simulink model "VSRMathematicalModel"  (R2021a)
settings: Solver=VariableStepAuto  StartTime=0.0  StopTime=0.3  FixedStep=5e-6  MaxStep=1e-6  RelTol=1e-3
InitFcn:
  | L = 2e-3;
  | omega = 2*pi*50;
  | a = exp(1i*2*pi/3);
  | R = 0.5;
  | C  = 1000e-6;
  | tau_c = 1.6e-4;
  | kp = L/tau_c;
  | ki = R/tau_c;
undefined symbols (not defined in the file): DiscIntNeverNeededParam
libraries: pid_lib x4
settings Model: Creator=Kibrom  LastModifiedBy=Kibrom

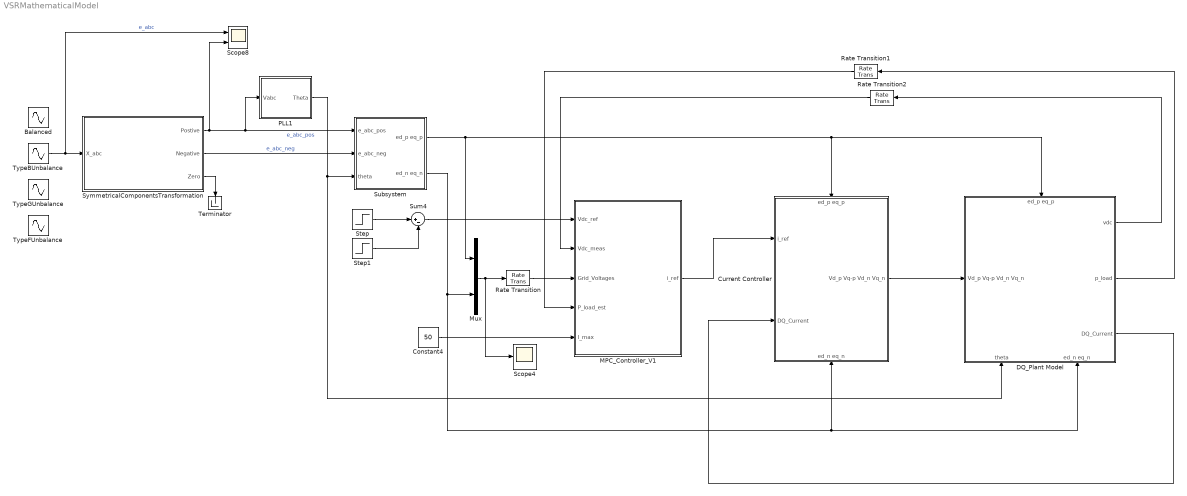
== system VSRMathematicalModel ==
  Balanced : Sin  Amplitude=sqrt(2)*[230 230 230]  Frequency=2*pi*50  Phase=[0 240 120]*(pi/180)  SampleTime=1e-4
  Constant4 : Constant  Value=50  SampleTime=1e-3
  Current Controller : Subsystem
      settings: PortSchema="{\"entries\":[{\"content\":{\"sides\":[{\"content\":{\"connectorIds\":[\"In1\",\"In2\"]},\"type\":\"ConnectorPlacement.EquallySpacedRectSide\",\"uuid\":\"d43164cf-c134-48fd-af5b-783b7be86266\"},{\"content\":{\"connectorIds\":[\"Out1\"],\"side\":\"RIGHT\"},\"type\":\"ConnectorPlacement.EquallySpacedRectSide\",\"uuid\":\"14eb066f-1df9-45e9-95e8-1c3f6be4e42a\"},{\"content\":{\"connectorIds\":[\"In3\"],\"side\":\"TOP\"},\"type\":\"ConnectorPlacement.EquallySpacedRectSide\",\"uuid\":\"0a2a25ed-4570-4f3f-83bf-cfa199df058c\"},{\"content\":{\"connectorIds\":[\"In4\"],\"side\":\"BOTTOM\"},\"type\":\"ConnectorPlacement.EquallySpacedRectSide\",\"uuid\":\"5d5e5ab5-6582-423d-8129-1371a7fc0364\"}]},\"type\":\"ConnectorPlacement.EquallySpacedConnector\",\"uuid\":\"cd9b7e71-8f1f-4781-be87-4737fe6c2517\"}],\"packageUris\":[\"http://schema.mathworks.com/mf0/Connector/R2020b\"],\"version\":\"1.0\"}"
  DQ_Plant Model : Subsystem
      settings: PortSchema="{\"entries\":[{\"content\":{\"sides\":[{\"content\":{\"connectorIds\":[\"In1\"]},\"type\":\"ConnectorPlacement.EquallySpacedRectSide\",\"uuid\":\"562d4ce7-556e-457d-bc10-9586690b759c\"},{\"content\":{\"connectorIds\":[\"Out1\",\"Out2\",\"Out3\"],\"side\":\"RIGHT\"},\"type\":\"ConnectorPlacement.EquallySpacedRectSide\",\"uuid\":\"d4e8a128-6870-4c36-a811-937c88534be6\"},{\"content\":{\"connectorIds\":[\"In2\"],\"side\":\"TOP\"},\"type\":\"ConnectorPlacement.EquallySpacedRectSide\",\"uuid\":\"ff397437-20b8-4b49-bf3a-8efc1e28b27f\"},{\"content\":{\"connectorIds\":[\"In3\",\"In4\"],\"side\":\"BOTTOM\"},\"type\":\"ConnectorPlacement.EquallySpacedRectSide\",\"uuid\":\"84aa63e1-bec8-4c80-97ac-aae86762ebfb\"}]},\"type\":\"ConnectorPlacement.EquallySpacedConnector\",\"uuid\":\"64a36633-d751-446b-85f3-9153f3d81120\"}],\"packageUris\":[\"http://schema.mathworks.com/mf0/Connector/R2020b\"],\"version\":\"1.0\"}"
  MPC_Controller_V1 : MATLAB Function  TreatAsAtomicUnit=on  SystemSampleTime=1e-3
  Mux : Mux  Inputs=2
  PLL1 : Subsystem
  Rate Transition : RateTransition  OutPortSampleTime=1000e-6
  Rate Transition1 : RateTransition
  Rate Transition2 : RateTransition
  Scope4 : Scope
  Scope8 : Scope  NumInputPorts=2
  Step : Step  Time=0.1  Before=650  After=750  SampleTime=1e-3
  Step1 : Step  Time=0.2  After=50  SampleTime=1e-3
  Subsystem : Subsystem
  Sum4 : Sum  Inputs=|+-
  SymmetricalComponentsTransformation : Subsystem
  Terminator : Terminator
  TypeBUnbalance : Sin  Amplitude=sqrt(2)*[185 230 230]  Frequency=2*pi*50  Phase=[0 240 120]*(pi/180)  SampleTime=0
  TypeFUnbalance : Sin  Amplitude=sqrt(2)*[184 207.4 207.4]  Frequency=2*pi*50  Phase=[0 243.7 116.3]*(pi/180)  SampleTime=0
  TypeGUnbalance : Sin  Amplitude=sqrt(2)*[214.6 192.1 192.1]  Frequency=2*pi*50  Phase=[0 236 124]*(pi/180)  SampleTime=0
  wires:
  SymmetricalComponentsTransformation/3(Zero) -> Terminator/1
  TypeBUnbalance/1 -> Scope8/1, SymmetricalComponentsTransformation/1(X_abc)  "e_abc"
  MPC_Controller_V1/1(i_ref) -> Current Controller/1(i_ref)
  Step/1 -> Sum4/1
  Mux/1 -> Scope4/1, Rate Transition/1
  Constant4/1 -> MPC_Controller_V1/5(I_max)
  Rate Transition/1 -> MPC_Controller_V1/3(Grid_Voltages)
  Rate Transition1/1 -> MPC_Controller_V1/4(P_load_est)
  Rate Transition2/1 -> MPC_Controller_V1/2(Vdc_meas)
  Step1/1 -> Sum4/2
  Sum4/1 -> MPC_Controller_V1/1(Vdc_ref)
  PLL1/1(Theta) -> Subsystem/3(theta), DQ_Plant Model/3(theta)
  SymmetricalComponentsTransformation/1(Postive) -> Scope8/2, Subsystem/1(e_abc_pos), PLL1/1(Vabc)  "e_abc_pos"
  Current Controller/1(Vd_p Vq-p Vd_n Vq_n) -> DQ_Plant Model/1(Vd_p Vq-p Vd_n Vq_n)
  DQ_Plant Model/1(vdc) -> Rate Transition2/1
  DQ_Plant Model/2(p_load) -> Rate Transition1/1
  DQ_Plant Model/3(DQ_Current) -> Current Controller/2(DQ_Current)
  Subsystem/1(ed_p eq_p) -> Mux/1, Current Controller/3(ed_p eq_p), DQ_Plant Model/2(ed_p eq_p)
  Subsystem/2(ed_n eq_n) -> Current Controller/4(ed_n eq_n), DQ_Plant Model/4(ed_n eq_n), Mux/2
  SymmetricalComponentsTransformation/2(Negative) -> Subsystem/2(e_abc_neg)  "e_abc_neg"

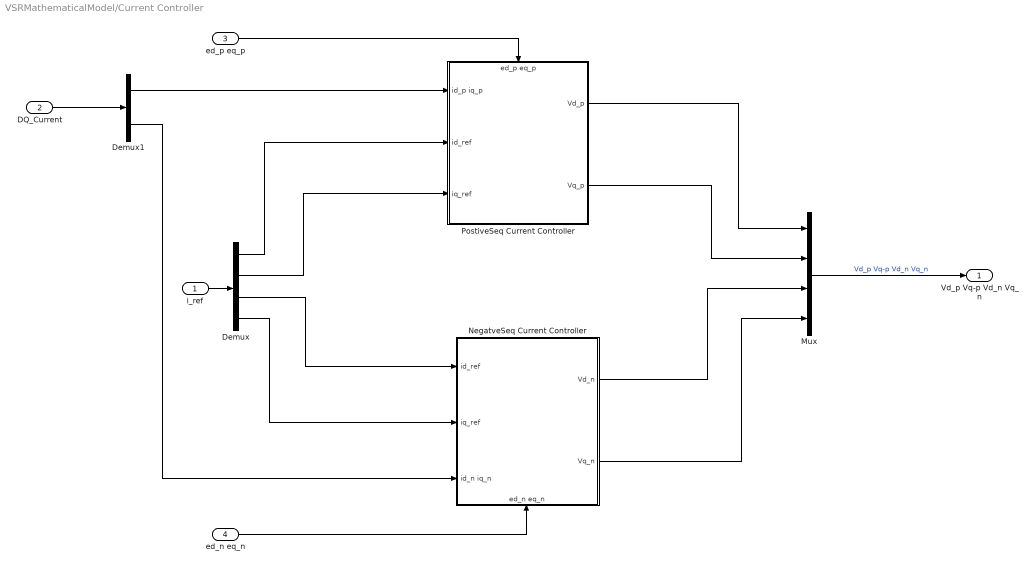
== system VSRMathematicalModel/Current Controller ==
  i_ref : Inport
  DQ_Current : Inport  Port=2
  ed_p eq_p : Inport  Port=3
  ed_n eq_n : Inport  Port=4
  Demux : Demux
  Demux1 : Demux  Outputs=2
  Mux : Mux
  NegatveSeq Current Controller : Subsystem
      settings: PortSchema="{\"entries\":[{\"content\":{\"sides\":[{\"content\":{\"connectorIds\":[\"In1\",\"In2\",\"In3\"]},\"type\":\"ConnectorPlacement.EquallySpacedRectSide\",\"uuid\":\"2bdf4aa8-c3f9-436b-9835-043d932fea71\"},{\"content\":{\"connectorIds\":[\"Out1\",\"Out2\"],\"side\":\"RIGHT\"},\"type\":\"ConnectorPlacement.EquallySpacedRectSide\",\"uuid\":\"c965a7a2-5936-47cc-8492-850bd324378e\"},{\"content\":{\"connectorIds\":[],\"side\":\"TOP\"},\"type\":\"ConnectorPlacement.EquallySpacedRectSide\",\"uuid\":\"45debca4-d3b7-48eb-be8d-4eccd646cb24\"},{\"content\":{\"connectorIds\":[\"In4\"],\"side\":\"BOTTOM\"},\"type\":\"ConnectorPlacement.EquallySpacedRectSide\",\"uuid\":\"6975aea9-83b3-4c6b-a4f1-94e60a0e1fe9\"}]},\"type\":\"ConnectorPlacement.EquallySpacedConnector\",\"uuid\":\"b897b5d1-f6c9-41b8-aee6-e6cc6417929b\"}],\"packageUris\":[\"http://schema.mathworks.com/mf0/Connector/R2020b\"],\"version\":\"1.0\"}"
  PostiveSeq Current Controller : Subsystem
      settings: PortSchema="{\"entries\":[{\"content\":{\"sides\":[{\"content\":{\"connectorIds\":[\"In1\",\"In2\",\"In3\"]},\"type\":\"ConnectorPlacement.EquallySpacedRectSide\",\"uuid\":\"2bdf4aa8-c3f9-436b-9835-043d932fea71\"},{\"content\":{\"connectorIds\":[\"Out1\",\"Out2\"],\"side\":\"RIGHT\"},\"type\":\"ConnectorPlacement.EquallySpacedRectSide\",\"uuid\":\"c965a7a2-5936-47cc-8492-850bd324378e\"},{\"content\":{\"connectorIds\":[\"In4\"],\"side\":\"TOP\"},\"type\":\"ConnectorPlacement.EquallySpacedRectSide\",\"uuid\":\"45debca4-d3b7-48eb-be8d-4eccd646cb24\"}]},\"type\":\"ConnectorPlacement.EquallySpacedConnector\",\"uuid\":\"b897b5d1-f6c9-41b8-aee6-e6cc6417929b\"}],\"packageUris\":[\"http://schema.mathworks.com/mf0/Connector/R2020b\"],\"version\":\"1.0\"}"
  Vd_p Vq-p Vd_n Vq_n : Outport
  wires:
  Demux1/1 -> PostiveSeq Current Controller/1(id_p iq_p)
  Demux/3 -> NegatveSeq Current Controller/1(id_ref)
  ed_n eq_n/1 -> NegatveSeq Current Controller/4(ed_n eq_n)
  PostiveSeq Current Controller/1(Vd_p) -> Mux/1
  ed_p eq_p/1 -> PostiveSeq Current Controller/4(ed_p eq_p)
  Demux/4 -> NegatveSeq Current Controller/2(iq_ref)
  NegatveSeq Current Controller/1(Vd_n) -> Mux/3
  NegatveSeq Current Controller/2(Vq_n) -> Mux/4
  Demux/1 -> PostiveSeq Current Controller/2(id_ref)
  Demux/2 -> PostiveSeq Current Controller/3(iq_ref)
  PostiveSeq Current Controller/2(Vq_p) -> Mux/2
  Demux1/2 -> NegatveSeq Current Controller/3(id_n iq_n)
  Mux/1 -> Vd_p Vq-p Vd_n Vq_n/1  "Vd_p Vq-p Vd_n Vq_n"
  i_ref/1 -> Demux/1
  DQ_Current/1 -> Demux1/1

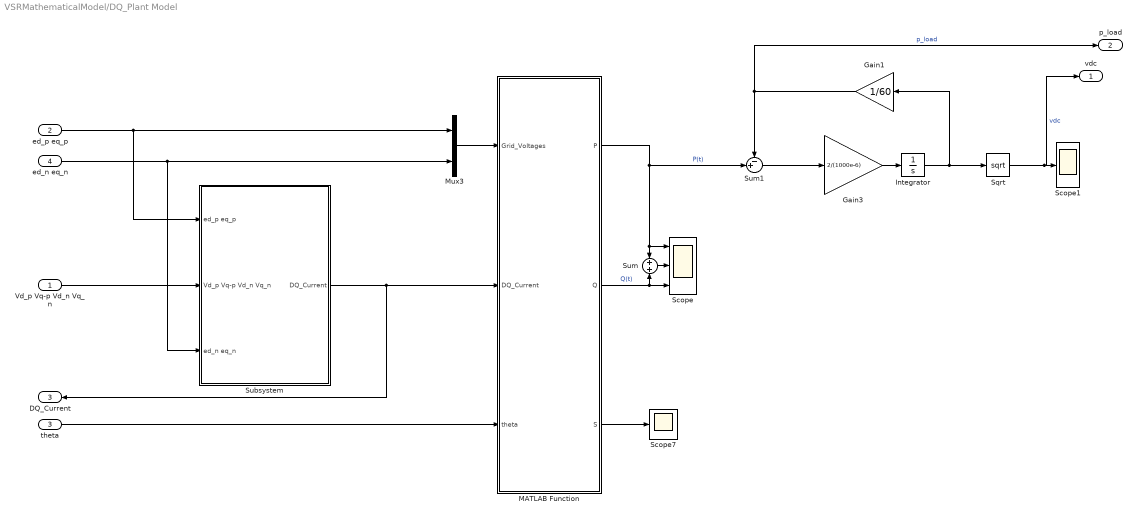
== system VSRMathematicalModel/DQ_Plant Model ==
  Vd_p Vq-p Vd_n Vq_n : Inport
  ed_p eq_p : Inport  Port=2
  theta : Inport  Port=3
  ed_n eq_n : Inport  Port=4
  Gain1 : Gain  Gain=1/60
  Gain3 : Gain  Gain=2/(1000e-6)
  Integrator : Integrator  InitialCondition=(650)^2
  MATLAB Function : MATLAB Function  TreatAsAtomicUnit=on
  Mux3 : Mux  Inputs=2
  Scope : Scope  NumInputPorts=3
  Scope1 : Scope
  Scope7 : Scope
  Sqrt : Sqrt  SaturateOnIntegerOverflow=on
  Subsystem : Subsystem
  Sum : Sum
  Sum1 : Sum  Inputs=-+|
  vdc : Outport
  p_load : Outport  Port=2
  DQ_Current : Outport  Port=3
  wires:
  MATLAB Function/3(S) -> Scope7/1
  Integrator/1 -> Sqrt/1, Gain1/1
  Gain1/1 -> p_load/1, Sum1/1  "p_load"
  ed_p eq_p/1 -> Subsystem/1(ed_p eq_p), Mux3/1
  MATLAB Function/2(Q) -> Scope/3, Sum/2  "Q(t)"
  Sum/1 -> Scope/2
  Gain3/1 -> Integrator/1
  MATLAB Function/1(P) -> Sum1/2, Scope/1, Sum/1  "P(t)"
  Sum1/1 -> Gain3/1
  Sqrt/1 -> vdc/1, Scope1/1  "vdc"
  ed_n eq_n/1 -> Subsystem/3(ed_n eq_n), Mux3/2
  Mux3/1 -> MATLAB Function/1(Grid_Voltages)
  Subsystem/1(DQ_Current) -> DQ_Current/1, MATLAB Function/2(DQ_Current)
  theta/1 -> MATLAB Function/3(theta)
  Vd_p Vq-p Vd_n Vq_n/1 -> Subsystem/2(Vd_p Vq-p Vd_n Vq_n)

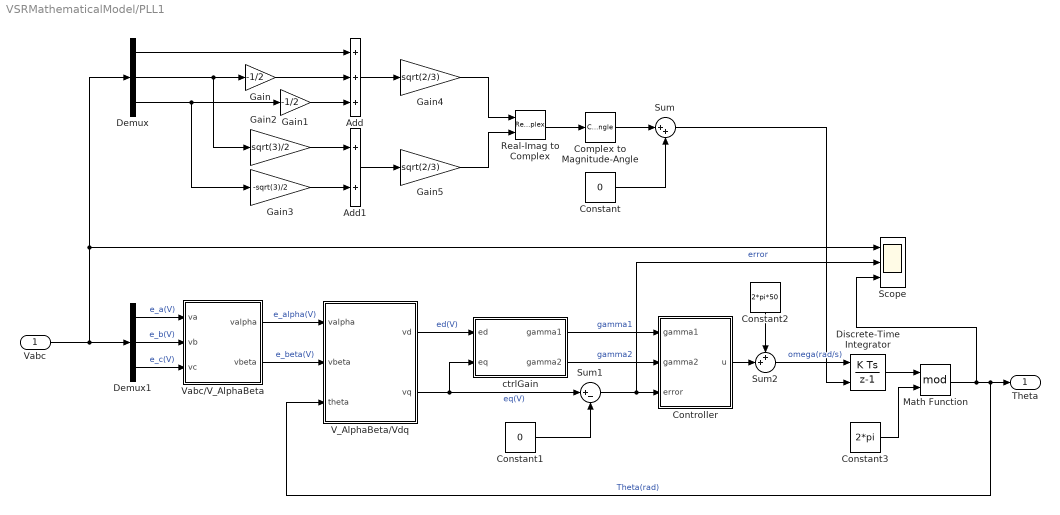
== system VSRMathematicalModel/PLL1 ==
  Vabc : Inport
  Add : Sum  Inputs=+++
  Add1 : Sum
  Complex to Magnitude-Angle : ComplexToMagnitudeAngle  Output=Angle
  Constant : Constant  Value=0
  Constant1 : Constant  Value=0
  Constant2 : Constant  Value=2*pi*50
  Constant3 : Constant  Value=2*pi
  Controller : Subsystem
  Demux : Demux  Outputs=3
  Demux1 : Demux  Outputs=3
  Discrete-Time Integrator : DiscreteIntegrator  InitialConditionSource=external  SampleTime=1e-4  ICPrevOutput=DiscIntNeverNeededParam  ICPrevScaledInput=DiscIntNeverNeededParam
  Gain : Gain  Gain=-1/2
  Gain1 : Gain  Gain=-1/2
  Gain2 : Gain  Gain=sqrt(3)/2
  Gain3 : Gain  Gain=-sqrt(3)/2
  Gain4 : Gain  Gain=sqrt(2/3)
  Gain5 : Gain  Gain=sqrt(2/3)
  Math Function : Math  Operator=mod  SaturateOnIntegerOverflow=on
  Real-Imag to Complex : RealImagToComplex
  Scope : Scope  NumInputPorts=3
  Sum : Sum  Inputs=|++
  Sum1 : Sum  Inputs=|+-
  Sum2 : Sum  Inputs=++|
  V_AlphaBeta/Vdq : MATLAB Function  TreatAsAtomicUnit=on
  Vabc/V_AlphaBeta : MATLAB Function  TreatAsAtomicUnit=on
  ctrlGain : MATLAB Function  TreatAsAtomicUnit=on
  Theta : Outport
  wires:
  Demux/2 -> Gain/1, Gain2/1
  Gain5/1 -> Real-Imag to Complex/2
  Add/1 -> Gain4/1
  Demux/3 -> Gain1/1, Gain3/1
  Gain/1 -> Add/2
  Gain4/1 -> Real-Imag to Complex/1
  Gain3/1 -> Add1/2
  Demux/1 -> Add/1
  Real-Imag to Complex/1 -> Complex to Magnitude-Angle/1
  Gain1/1 -> Add/3
  Add1/1 -> Gain5/1
  Gain2/1 -> Add1/1
  Complex to Magnitude-Angle/1 -> Sum/1
  Sum/1 -> Discrete-Time Integrator/2
  Constant/1 -> Sum/2
  Demux1/2 -> Vabc/V_AlphaBeta/2(vb)  "e_b(V)"
  Demux1/3 -> Vabc/V_AlphaBeta/3(vc)  "e_c(V)"
  Demux1/1 -> Vabc/V_AlphaBeta/1(va)  "e_a(V)"
  Vabc/V_AlphaBeta/2(vbeta) -> V_AlphaBeta/Vdq/2(vbeta)  "e_beta(V)"
  Vabc/V_AlphaBeta/1(valpha) -> V_AlphaBeta/Vdq/1(valpha)  "e_alpha(V)"
  V_AlphaBeta/Vdq/2(vq) -> ctrlGain/2(eq), Sum1/1  "eq(V)"
  Constant1/1 -> Sum1/2
  Constant2/1 -> Sum2/1
  Sum2/1 -> Discrete-Time Integrator/1  "omega(rad/s)"
  Discrete-Time Integrator/1 -> Math Function/1
  V_AlphaBeta/Vdq/1(vd) -> ctrlGain/1(ed)  "ed(V)"
  ctrlGain/1(gamma1) -> Controller/1(gamma1)  "gamma1"
  ctrlGain/2(gamma2) -> Controller/2(gamma2)  "gamma2"
  Sum1/1 -> Scope/2, Controller/3(error)  "error"
  Controller/1(u) -> Sum2/2
  Math Function/1 -> Scope/3, Theta/1, V_AlphaBeta/Vdq/3(theta)  "Theta(rad)"
  Constant3/1 -> Math Function/2
  Vabc/1 -> Demux/1, Scope/1, Demux1/1

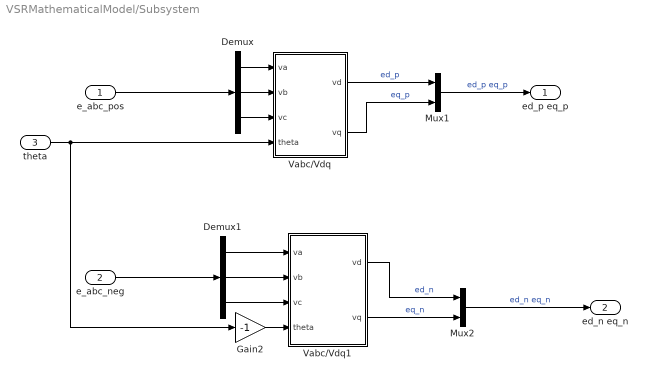
== system VSRMathematicalModel/Subsystem ==
  e_abc_pos : Inport
  e_abc_neg : Inport  Port=2
  theta : Inport  Port=3
  Demux : Demux  Outputs=3
  Demux1 : Demux  Outputs=3
  Gain2 : Gain  Gain=-1
  Mux1 : Mux  Inputs=2
  Mux2 : Mux  Inputs=2
  Vabc/Vdq : MATLAB Function  TreatAsAtomicUnit=on
  Vabc/Vdq1 : MATLAB Function  TreatAsAtomicUnit=on
  ed_p eq_p : Outport
  ed_n eq_n : Outport  Port=2
  wires:
  Vabc/Vdq1/2(vq) -> Mux2/2  "eq_n"
  Demux/1 -> Vabc/Vdq/1(va)
  Vabc/Vdq/1(vd) -> Mux1/1  "ed_p"
  Demux/2 -> Vabc/Vdq/2(vb)
  Demux1/3 -> Vabc/Vdq1/3(vc)
  Vabc/Vdq1/1(vd) -> Mux2/1  "ed_n"
  Demux1/2 -> Vabc/Vdq1/2(vb)
  Vabc/Vdq/2(vq) -> Mux1/2  "eq_p"
  e_abc_pos/1 -> Demux/1
  Demux1/1 -> Vabc/Vdq1/1(va)
  Gain2/1 -> Vabc/Vdq1/4(theta)
  Demux/3 -> Vabc/Vdq/3(vc)
  Mux1/1 -> ed_p eq_p/1  "ed_p eq_p"
  Mux2/1 -> ed_n eq_n/1  "ed_n eq_n"
  theta/1 -> Gain2/1, Vabc/Vdq/4(theta)
  e_abc_neg/1 -> Demux1/1

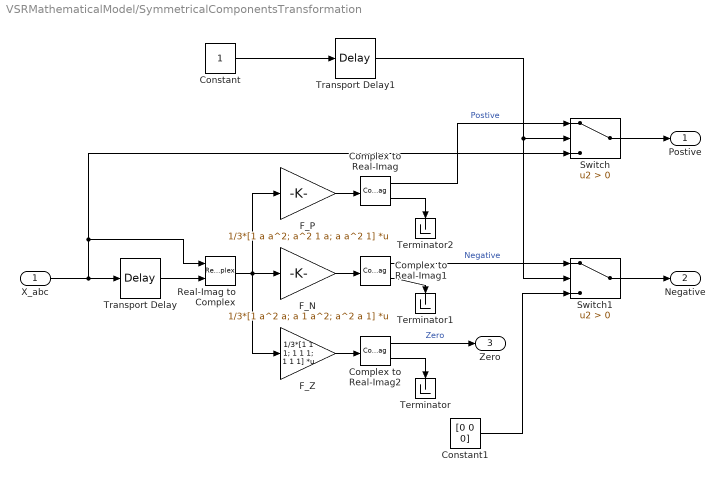
== system VSRMathematicalModel/SymmetricalComponentsTransformation ==
  X_abc : Inport
  Complex to Real-Imag : ComplexToRealImag
  Complex to Real-Imag1 : ComplexToRealImag
  Complex to Real-Imag2 : ComplexToRealImag
  Constant : Constant
  Constant1 : Constant  Value=[0 0 0]
  F_N : Gain  Gain=1/3*[1 a^2 a; a 1 a^2; a^2 a 1]  Multiplication=Matrix(K*u)
  F_P : Gain  Gain=1/3*[1 a a^2; a^2 1 a; a a^2 1]  Multiplication=Matrix(K*u)
  F_Z : Gain  Gain=1/3*[1 1 1; 1 1 1; 1 1 1]  Multiplication=Matrix(K*u)
  Real-Imag to Complex : RealImagToComplex
  Switch : Switch  Criteria=u2 > Threshold
  Switch1 : Switch  Criteria=u2 > Threshold
  Terminator : Terminator
  Terminator1 : Terminator
  Terminator2 : Terminator
  Transport Delay : TransportDelay  DelayTime=1/(4*50)  BufferSize=10000
  Transport Delay1 : TransportDelay  DelayTime=1/(4*50)  BufferSize=10000
  Postive : Outport
  Negative : Outport  Port=2
  Zero : Outport  Port=3
  wires:
  Constant1/1 -> Switch1/3
  Complex to Real-Imag1/1 -> Switch1/1  "Negative"
  Switch1/1 -> Negative/1
  Transport Delay/1 -> Real-Imag to Complex/2
  Real-Imag to Complex/1 -> F_P/1, F_Z/1, F_N/1
  Complex to Real-Imag2/2 -> Terminator/1
  F_Z/1 -> Complex to Real-Imag2/1
  Switch/1 -> Postive/1
  Constant/1 -> Transport Delay1/1
  Complex to Real-Imag2/1 -> Zero/1  "Zero"
  Transport Delay1/1 -> Switch1/2, Switch/2
  F_P/1 -> Complex to Real-Imag/1
  F_N/1 -> Complex to Real-Imag1/1
  Complex to Real-Imag1/2 -> Terminator1/1
  X_abc/1 -> Real-Imag to Complex/1, Switch/3, Transport Delay/1
  Complex to Real-Imag/1 -> Switch/1  "Postive"
  Complex to Real-Imag/2 -> Terminator2/1

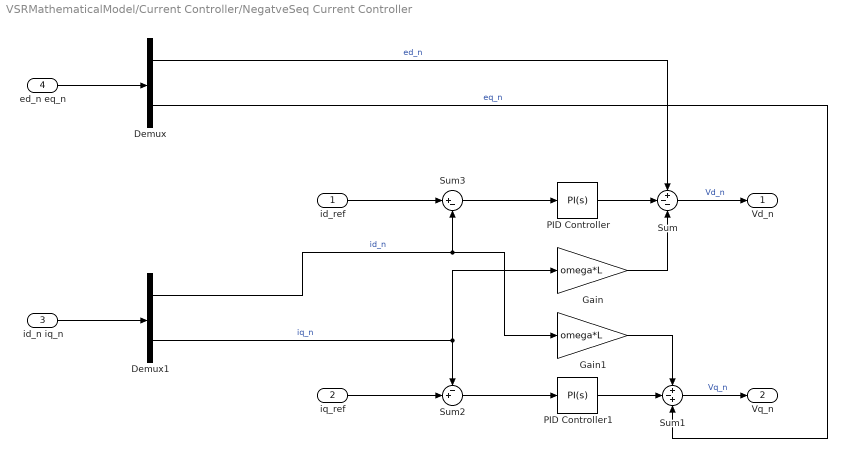
== system VSRMathematicalModel/Current Controller/NegatveSeq Current Controller ==
  id_ref : Inport
  iq_ref : Inport  Port=2
  id_n iq_n : Inport  Port=3
  ed_n eq_n : Inport  Port=4
  Demux : Demux  Outputs=2
  Demux1 : Demux  Outputs=2
  Gain : Gain  Gain=omega*L
  Gain1 : Gain  Gain=omega*L
  PID Controller : pid_lib/PID Controller  Controller=PI  Form=Parallel  TimeDomain=Continuous-time  UseExternalTs=off  SampleTime=-1  IntegratorMethod=Forward Euler  FilterMethod=Forward Euler  ControllerParametersSource=internal  P=kp  I=ki  D=0  UseFilter=on  N=100  TunerSelectOption=Transfer Function Based (PID Tuner App)  InitialConditionSource=internal  InitialConditionForIntegrator=0  InitialConditionForFilter=0  DifferentiatorICPrevScaledInput=0  ExternalReset=none  TrackingMode=off  Kt=1  LimitOutput=off  SatLimitsSource=internal  UpperSaturationLimit=inf  LowerSaturationLimit=-inf  LinearizeAsGain=on  AntiWindupMode=none  Kb=1  POutMin=[]  POutMax=[]  IOutMin=[]  IOutMax=[]  DOutMin=[]  DOutMax=[]  NOutMin=[]  NOutMax=[]  SumOutMin=[]  SumOutMax=[]  SaturationOutMin=[]  SaturationOutMax=[]  PParamMin=[]  PParamMax=[]  IParamMin=[]  IParamMax=[]  DParamMin=[]  DParamMax=[]  NParamMin=[]  NParamMax=[]  KbParamMin=[]  KbParamMax=[]  KtParamMin=[]  KtParamMax=[]  KbOutMin=[]  KbOutMax=[]  KtOutMin=[]  KtOutMax=[]  IntegratorOutMin=[]  IntegratorOutMax=[]  FilterOutMin=[]  FilterOutMax=[]  SumI1OutMin=[]  SumI1OutMax=[]  SumI2OutMin=[]  SumI2OutMax=[]  SumI3OutMin=[]  SumI3OutMax=[]  SumI4OutMin=[]  SumI4OutMax=[]  SumDOutMin=[]  SumDOutMax=[]  DifferentiatorOutMin=[]  DifferentiatorOutMax=[]  FilterDiffOutCoefMin=[]  FilterDiffOutCoefMax=[]  ReciprocalOutMin=[]  ReciprocalOutMax=[]  SumDenOutMin=[]  SumDenOutMax=[]  SumNumOutMin=[]  SumNumOutMax=[]  DivideOutMin=[]  DivideOutMax=[]  UdiffTsProdOutMin=[]  UdiffTsProdOutMax=[]  NTsProdOutMin=[]  NTsProdOutMax=[]  UintegralTsProdOutMin=[]  UintegralTsProdOutMax=[]  UngainTsProdOutMin=[]  UngainTsProdOutMax=[]  IntegratorContinuousStateAttributes=''  IntegratorStateMustResolveToSignalObject=off  IntegratorRTWStateStorageClass=Auto  FilterContinuousStateAttributes=''  FilterStateMustResolveToSignalObject=off  FilterRTWStateStorageClass=Auto  ParallelPVariant=InternalParameters  IdealPVariant=Disabled  IVariant=InternalParameters  DVariant=Disabled  IntegratorVariant=Continuous  SatVariant=Disabled  AWVariant=Passthrough  PCopyVariant=Disabled  TRVariant=Disabled  FdbkBlocksVariant=Forward  IdealPFdbkVariant=Disabled  SatFdbkVariant=Disabled  DerivativeFilterVariant=Disabled  NVariant=Disabled  NCopyVariant=Disabled_SignalSpec  FilterICVariant=Disabled  IntegratorICVariant=InternalICs  ExternalResetVariant=Disabled  TRSumVariant=Passthrough  SumFdbkVariant=Disabled  SumVariant=Sum_PI  TsampFilterVariant=InternalTs  TsampNgainVariant=Passthrough  TsampIntegralVariant=Passthrough  ExternalSaturationOutDataTypeStr=Inherit: Same as second input
  PID Controller1 : pid_lib/PID Controller  Controller=PI  Form=Parallel  TimeDomain=Continuous-time  UseExternalTs=off  SampleTime=-1  IntegratorMethod=Forward Euler  FilterMethod=Forward Euler  ControllerParametersSource=internal  P=kp  I=ki  D=0  UseFilter=on  N=100  TunerSelectOption=Transfer Function Based (PID Tuner App)  InitialConditionSource=internal  InitialConditionForIntegrator=0  InitialConditionForFilter=0  DifferentiatorICPrevScaledInput=0  ExternalReset=none  TrackingMode=off  Kt=1  LimitOutput=off  SatLimitsSource=internal  UpperSaturationLimit=inf  LowerSaturationLimit=-inf  LinearizeAsGain=on  AntiWindupMode=none  Kb=1  POutMin=[]  POutMax=[]  IOutMin=[]  IOutMax=[]  DOutMin=[]  DOutMax=[]  NOutMin=[]  NOutMax=[]  SumOutMin=[]  SumOutMax=[]  SaturationOutMin=[]  SaturationOutMax=[]  PParamMin=[]  PParamMax=[]  IParamMin=[]  IParamMax=[]  DParamMin=[]  DParamMax=[]  NParamMin=[]  NParamMax=[]  KbParamMin=[]  KbParamMax=[]  KtParamMin=[]  KtParamMax=[]  KbOutMin=[]  KbOutMax=[]  KtOutMin=[]  KtOutMax=[]  IntegratorOutMin=[]  IntegratorOutMax=[]  FilterOutMin=[]  FilterOutMax=[]  SumI1OutMin=[]  SumI1OutMax=[]  SumI2OutMin=[]  SumI2OutMax=[]  SumI3OutMin=[]  SumI3OutMax=[]  SumI4OutMin=[]  SumI4OutMax=[]  SumDOutMin=[]  SumDOutMax=[]  DifferentiatorOutMin=[]  DifferentiatorOutMax=[]  FilterDiffOutCoefMin=[]  FilterDiffOutCoefMax=[]  ReciprocalOutMin=[]  ReciprocalOutMax=[]  SumDenOutMin=[]  SumDenOutMax=[]  SumNumOutMin=[]  SumNumOutMax=[]  DivideOutMin=[]  DivideOutMax=[]  UdiffTsProdOutMin=[]  UdiffTsProdOutMax=[]  NTsProdOutMin=[]  NTsProdOutMax=[]  UintegralTsProdOutMin=[]  UintegralTsProdOutMax=[]  UngainTsProdOutMin=[]  UngainTsProdOutMax=[]  IntegratorContinuousStateAttributes=''  IntegratorStateMustResolveToSignalObject=off  IntegratorRTWStateStorageClass=Auto  FilterContinuousStateAttributes=''  FilterStateMustResolveToSignalObject=off  FilterRTWStateStorageClass=Auto  ParallelPVariant=InternalParameters  IdealPVariant=Disabled  IVariant=InternalParameters  DVariant=Disabled  IntegratorVariant=Continuous  SatVariant=Disabled  AWVariant=Passthrough  PCopyVariant=Disabled  TRVariant=Disabled  FdbkBlocksVariant=Forward  IdealPFdbkVariant=Disabled  SatFdbkVariant=Disabled  DerivativeFilterVariant=Disabled  NVariant=Disabled  NCopyVariant=Disabled_SignalSpec  FilterICVariant=Disabled  IntegratorICVariant=InternalICs  ExternalResetVariant=Disabled  TRSumVariant=Passthrough  SumFdbkVariant=Disabled  SumVariant=Sum_PI  TsampFilterVariant=InternalTs  TsampNgainVariant=Passthrough  TsampIntegralVariant=Passthrough  ExternalSaturationOutDataTypeStr=Inherit: Same as second input
  Sum : Sum  Inputs=+--
  Sum1 : Sum  Inputs=+-+
  Sum2 : Sum  Inputs=-+|
  Sum3 : Sum  Inputs=|+-
  Vd_n : Outport
  Vq_n : Outport  Port=2
  wires:
  Sum/1 -> Vd_n/1  "Vd_n"
  Sum1/1 -> Vq_n/1  "Vq_n"
  id_ref/1 -> Sum3/1
  Sum3/1 -> PID Controller/1
  iq_ref/1 -> Sum2/2
  Demux/1 -> Sum/1  "ed_n"
  Gain1/1 -> Sum1/1
  PID Controller/1 -> Sum/2
  PID Controller1/1 -> Sum1/2
  Gain/1 -> Sum/3
  Sum2/1 -> PID Controller1/1
  Demux/2 -> Sum1/3  "eq_n"
  ed_n eq_n/1 -> Demux/1
  id_n iq_n/1 -> Demux1/1
  Demux1/2 -> Gain/1, Sum2/1  "iq_n"
  Demux1/1 -> Gain1/1, Sum3/2  "id_n"

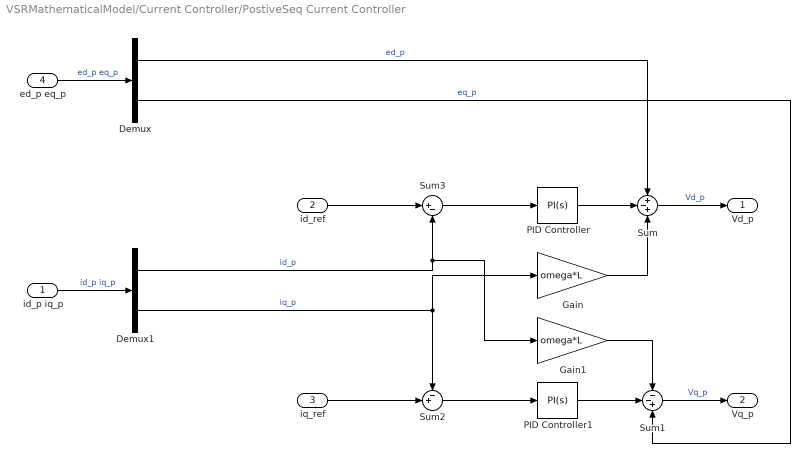
== system VSRMathematicalModel/Current Controller/PostiveSeq Current Controller ==
  id_p iq_p : Inport
  id_ref : Inport  Port=2
  iq_ref : Inport  Port=3
  ed_p eq_p : Inport  Port=4
  Demux : Demux  Outputs=2
  Demux1 : Demux  Outputs=2
  Gain : Gain  Gain=omega*L
  Gain1 : Gain  Gain=omega*L
  PID Controller : pid_lib/PID Controller  Controller=PI  Form=Parallel  TimeDomain=Continuous-time  UseExternalTs=off  SampleTime=-1  IntegratorMethod=Forward Euler  FilterMethod=Forward Euler  ControllerParametersSource=internal  P=kp  I=ki  D=0  UseFilter=on  N=100  TunerSelectOption=Transfer Function Based (PID Tuner App)  InitialConditionSource=internal  InitialConditionForIntegrator=0  InitialConditionForFilter=0  DifferentiatorICPrevScaledInput=0  ExternalReset=none  TrackingMode=off  Kt=1  LimitOutput=off  SatLimitsSource=internal  UpperSaturationLimit=inf  LowerSaturationLimit=-inf  LinearizeAsGain=on  AntiWindupMode=none  Kb=1  POutMin=[]  POutMax=[]  IOutMin=[]  IOutMax=[]  DOutMin=[]  DOutMax=[]  NOutMin=[]  NOutMax=[]  SumOutMin=[]  SumOutMax=[]  SaturationOutMin=[]  SaturationOutMax=[]  PParamMin=[]  PParamMax=[]  IParamMin=[]  IParamMax=[]  DParamMin=[]  DParamMax=[]  NParamMin=[]  NParamMax=[]  KbParamMin=[]  KbParamMax=[]  KtParamMin=[]  KtParamMax=[]  KbOutMin=[]  KbOutMax=[]  KtOutMin=[]  KtOutMax=[]  IntegratorOutMin=[]  IntegratorOutMax=[]  FilterOutMin=[]  FilterOutMax=[]  SumI1OutMin=[]  SumI1OutMax=[]  SumI2OutMin=[]  SumI2OutMax=[]  SumI3OutMin=[]  SumI3OutMax=[]  SumI4OutMin=[]  SumI4OutMax=[]  SumDOutMin=[]  SumDOutMax=[]  DifferentiatorOutMin=[]  DifferentiatorOutMax=[]  FilterDiffOutCoefMin=[]  FilterDiffOutCoefMax=[]  ReciprocalOutMin=[]  ReciprocalOutMax=[]  SumDenOutMin=[]  SumDenOutMax=[]  SumNumOutMin=[]  SumNumOutMax=[]  DivideOutMin=[]  DivideOutMax=[]  UdiffTsProdOutMin=[]  UdiffTsProdOutMax=[]  NTsProdOutMin=[]  NTsProdOutMax=[]  UintegralTsProdOutMin=[]  UintegralTsProdOutMax=[]  UngainTsProdOutMin=[]  UngainTsProdOutMax=[]  IntegratorContinuousStateAttributes=''  IntegratorStateMustResolveToSignalObject=off  IntegratorRTWStateStorageClass=Auto  FilterContinuousStateAttributes=''  FilterStateMustResolveToSignalObject=off  FilterRTWStateStorageClass=Auto  ParallelPVariant=InternalParameters  IdealPVariant=Disabled  IVariant=InternalParameters  DVariant=Disabled  IntegratorVariant=Continuous  SatVariant=Disabled  AWVariant=Passthrough  PCopyVariant=Disabled  TRVariant=Disabled  FdbkBlocksVariant=Forward  IdealPFdbkVariant=Disabled  SatFdbkVariant=Disabled  DerivativeFilterVariant=Disabled  NVariant=Disabled  NCopyVariant=Disabled_SignalSpec  FilterICVariant=Disabled  IntegratorICVariant=InternalICs  ExternalResetVariant=Disabled  TRSumVariant=Passthrough  SumFdbkVariant=Disabled  SumVariant=Sum_PI  TsampFilterVariant=InternalTs  TsampNgainVariant=Passthrough  TsampIntegralVariant=Passthrough  ExternalSaturationOutDataTypeStr=Inherit: Same as second input
  PID Controller1 : pid_lib/PID Controller  Controller=PI  Form=Parallel  TimeDomain=Continuous-time  UseExternalTs=off  SampleTime=-1  IntegratorMethod=Forward Euler  FilterMethod=Forward Euler  ControllerParametersSource=internal  P=kp  I=ki  D=0  UseFilter=on  N=100  TunerSelectOption=Transfer Function Based (PID Tuner App)  InitialConditionSource=internal  InitialConditionForIntegrator=0  InitialConditionForFilter=0  DifferentiatorICPrevScaledInput=0  ExternalReset=none  TrackingMode=off  Kt=1  LimitOutput=off  SatLimitsSource=internal  UpperSaturationLimit=inf  LowerSaturationLimit=-inf  LinearizeAsGain=on  AntiWindupMode=none  Kb=1  POutMin=[]  POutMax=[]  IOutMin=[]  IOutMax=[]  DOutMin=[]  DOutMax=[]  NOutMin=[]  NOutMax=[]  SumOutMin=[]  SumOutMax=[]  SaturationOutMin=[]  SaturationOutMax=[]  PParamMin=[]  PParamMax=[]  IParamMin=[]  IParamMax=[]  DParamMin=[]  DParamMax=[]  NParamMin=[]  NParamMax=[]  KbParamMin=[]  KbParamMax=[]  KtParamMin=[]  KtParamMax=[]  KbOutMin=[]  KbOutMax=[]  KtOutMin=[]  KtOutMax=[]  IntegratorOutMin=[]  IntegratorOutMax=[]  FilterOutMin=[]  FilterOutMax=[]  SumI1OutMin=[]  SumI1OutMax=[]  SumI2OutMin=[]  SumI2OutMax=[]  SumI3OutMin=[]  SumI3OutMax=[]  SumI4OutMin=[]  SumI4OutMax=[]  SumDOutMin=[]  SumDOutMax=[]  DifferentiatorOutMin=[]  DifferentiatorOutMax=[]  FilterDiffOutCoefMin=[]  FilterDiffOutCoefMax=[]  ReciprocalOutMin=[]  ReciprocalOutMax=[]  SumDenOutMin=[]  SumDenOutMax=[]  SumNumOutMin=[]  SumNumOutMax=[]  DivideOutMin=[]  DivideOutMax=[]  UdiffTsProdOutMin=[]  UdiffTsProdOutMax=[]  NTsProdOutMin=[]  NTsProdOutMax=[]  UintegralTsProdOutMin=[]  UintegralTsProdOutMax=[]  UngainTsProdOutMin=[]  UngainTsProdOutMax=[]  IntegratorContinuousStateAttributes=''  IntegratorStateMustResolveToSignalObject=off  IntegratorRTWStateStorageClass=Auto  FilterContinuousStateAttributes=''  FilterStateMustResolveToSignalObject=off  FilterRTWStateStorageClass=Auto  ParallelPVariant=InternalParameters  IdealPVariant=Disabled  IVariant=InternalParameters  DVariant=Disabled  IntegratorVariant=Continuous  SatVariant=Disabled  AWVariant=Passthrough  PCopyVariant=Disabled  TRVariant=Disabled  FdbkBlocksVariant=Forward  IdealPFdbkVariant=Disabled  SatFdbkVariant=Disabled  DerivativeFilterVariant=Disabled  NVariant=Disabled  NCopyVariant=Disabled_SignalSpec  FilterICVariant=Disabled  IntegratorICVariant=InternalICs  ExternalResetVariant=Disabled  TRSumVariant=Passthrough  SumFdbkVariant=Disabled  SumVariant=Sum_PI  TsampFilterVariant=InternalTs  TsampNgainVariant=Passthrough  TsampIntegralVariant=Passthrough  ExternalSaturationOutDataTypeStr=Inherit: Same as second input
  Sum : Sum  Inputs=+-+
  Sum1 : Sum  Inputs=--+
  Sum2 : Sum  Inputs=-+|
  Sum3 : Sum  Inputs=|+-
  Vd_p : Outport
  Vq_p : Outport  Port=2
  wires:
  Demux/2 -> Sum1/3  "eq_p"
  Sum2/1 -> PID Controller1/1
  Gain/1 -> Sum/3
  PID Controller1/1 -> Sum1/2
  PID Controller/1 -> Sum/2
  Gain1/1 -> Sum1/1
  Demux/1 -> Sum/1  "ed_p"
  iq_ref/1 -> Sum2/2
  Sum3/1 -> PID Controller/1
  id_ref/1 -> Sum3/1
  Sum1/1 -> Vq_p/1  "Vq_p"
  Sum/1 -> Vd_p/1  "Vd_p"
  ed_p eq_p/1 -> Demux/1  "ed_p eq_p"
  Demux1/2 -> Gain/1, Sum2/1  "iq_p"
  Demux1/1 -> Sum3/2, Gain1/1  "id_p"
  id_p iq_p/1 -> Demux1/1  "id_p iq_p"

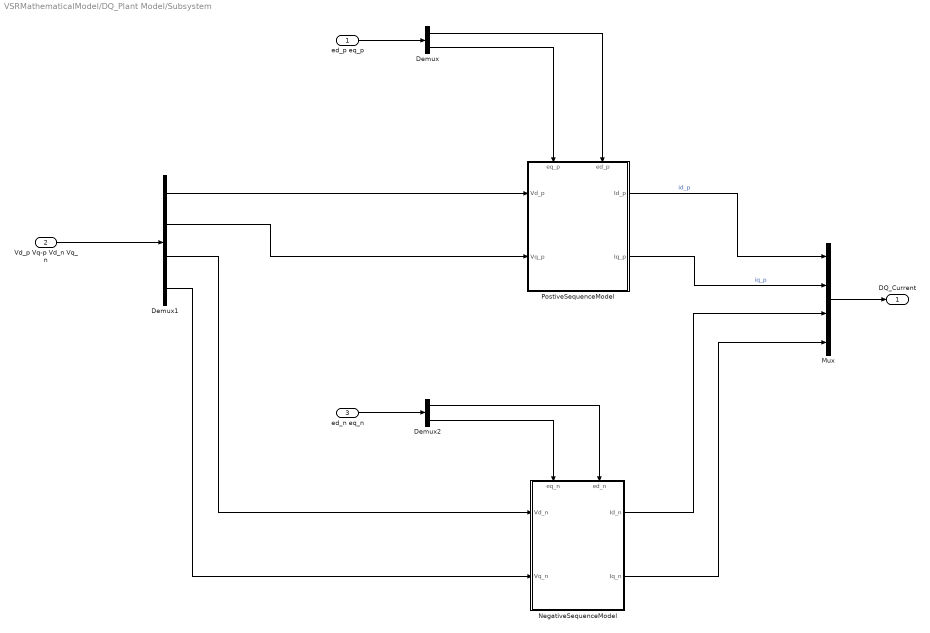
== system VSRMathematicalModel/DQ_Plant Model/Subsystem ==
  ed_p eq_p : Inport
  Vd_p Vq-p Vd_n Vq_n : Inport  Port=2
  ed_n eq_n : Inport  Port=3
  Demux : Demux  Outputs=2
  Demux1 : Demux
  Demux2 : Demux  Outputs=2
  Mux : Mux
  NegativeSequenceModel : Subsystem
      settings: PortSchema="{\"entries\":[{\"content\":{\"sides\":[{\"content\":{\"connectorIds\":[\"In1\",\"In2\"]},\"type\":\"ConnectorPlacement.EquallySpacedRectSide\",\"uuid\":\"35b4db01-9104-4f8b-8b75-246466a1ebf9\"},{\"content\":{\"connectorIds\":[\"Out1\",\"Out2\"],\"side\":\"RIGHT\"},\"type\":\"ConnectorPlacement.EquallySpacedRectSide\",\"uuid\":\"71a10765-5020-4c51-b6ed-4b6513a95dba\"},{\"content\":{\"connectorIds\":[\"In3\",\"In4\"],\"side\":\"TOP\"},\"type\":\"ConnectorPlacement.EquallySpacedRectSide\",\"uuid\":\"61c862d8-7219-4ead-87db-e5ab0ab1f151\"}]},\"type\":\"ConnectorPlacement.EquallySpacedConnector\",\"uuid\":\"950d7f7d-ddec-4099-934f-f7ca3b417813\"}],\"packageUris\":[\"http://schema.mathworks.com/mf0/Connector/R2020b\"],\"version\":\"1.0\"}"
  PostiveSequenceModel : Subsystem
      settings: PortSchema="{\"entries\":[{\"content\":{\"sides\":[{\"content\":{\"connectorIds\":[\"In1\",\"In2\"]},\"type\":\"ConnectorPlacement.EquallySpacedRectSide\",\"uuid\":\"35b4db01-9104-4f8b-8b75-246466a1ebf9\"},{\"content\":{\"connectorIds\":[\"Out1\",\"Out2\"],\"side\":\"RIGHT\"},\"type\":\"ConnectorPlacement.EquallySpacedRectSide\",\"uuid\":\"71a10765-5020-4c51-b6ed-4b6513a95dba\"},{\"content\":{\"connectorIds\":[\"In3\",\"In4\"],\"side\":\"TOP\"},\"type\":\"ConnectorPlacement.EquallySpacedRectSide\",\"uuid\":\"61c862d8-7219-4ead-87db-e5ab0ab1f151\"}]},\"type\":\"ConnectorPlacement.EquallySpacedConnector\",\"uuid\":\"950d7f7d-ddec-4099-934f-f7ca3b417813\"}],\"packageUris\":[\"http://schema.mathworks.com/mf0/Connector/R2020b\"],\"version\":\"1.0\"}"
  DQ_Current : Outport
  wires:
  PostiveSequenceModel/2(Iq_p) -> Mux/2  "iq_p"
  Demux2/2 -> NegativeSequenceModel/3(eq_n)
  Demux1/2 -> PostiveSequenceModel/2(Vq_p)
  NegativeSequenceModel/2(Iq_n) -> Mux/4
  PostiveSequenceModel/1(Id_p) -> Mux/1  "id_p"
  NegativeSequenceModel/1(Id_n) -> Mux/3
  Demux1/1 -> PostiveSequenceModel/1(Vd_p)
  Demux2/1 -> NegativeSequenceModel/4(ed_n)
  Demux/1 -> PostiveSequenceModel/4(ed_p)
  Demux/2 -> PostiveSequenceModel/3(eq_p)
  ed_p eq_p/1 -> Demux/1
  Vd_p Vq-p Vd_n Vq_n/1 -> Demux1/1
  Demux1/3 -> NegativeSequenceModel/1(Vd_n)
  Demux1/4 -> NegativeSequenceModel/2(Vq_n)
  ed_n eq_n/1 -> Demux2/1
  Mux/1 -> DQ_Current/1

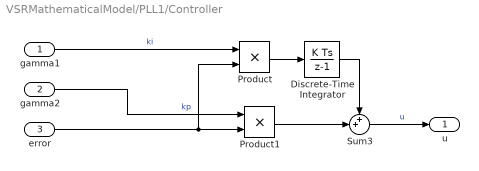
== system VSRMathematicalModel/PLL1/Controller ==
  gamma1 : Inport
  gamma2 : Inport  Port=2
  error : Inport  Port=3
  Discrete-Time Integrator : DiscreteIntegrator  SampleTime=1e-4  ICPrevOutput=DiscIntNeverNeededParam  ICPrevScaledInput=DiscIntNeverNeededParam
  Product : Product
  Product1 : Product
  Sum3 : Sum  Inputs=++|
  u : Outport
  wires:
  Product1/1 -> Sum3/2
  Product/1 -> Discrete-Time Integrator/1
  error/1 -> Product1/2, Product/2
  gamma2/1 -> Product1/1  "kp"
  Sum3/1 -> u/1  "u"
  Discrete-Time Integrator/1 -> Sum3/1
  gamma1/1 -> Product/1  "ki"

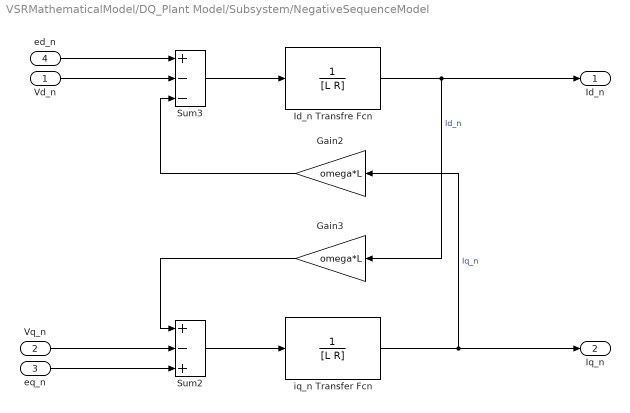
== system VSRMathematicalModel/DQ_Plant Model/Subsystem/NegativeSequenceModel ==
  Vd_n : Inport
  Vq_n : Inport  Port=2
  eq_n : Inport  Port=3
  ed_n : Inport  Port=4
  Gain2 : Gain  Gain=omega*L
  Gain3 : Gain  Gain=omega*L
  Id_n Transfre Fcn : TransferFcn  Denominator=[L R]
  Sum2 : Sum  Inputs=+-+
  Sum3 : Sum  Inputs=+--
  iq_n Transfer Fcn : TransferFcn  Denominator=[L R]
  Id_n : Outport
  Iq_n : Outport  Port=2
  wires:
  eq_n/1 -> Sum2/3
  Sum3/1 -> Id_n Transfre Fcn/1
  Id_n Transfre Fcn/1 -> Id_n/1, Gain3/1  "Id_n"
  Sum2/1 -> iq_n Transfer Fcn/1
  Gain2/1 -> Sum3/3
  Vd_n/1 -> Sum3/2
  Gain3/1 -> Sum2/1
  iq_n Transfer Fcn/1 -> Iq_n/1, Gain2/1  "Iq_n"
  ed_n/1 -> Sum3/1
  Vq_n/1 -> Sum2/2

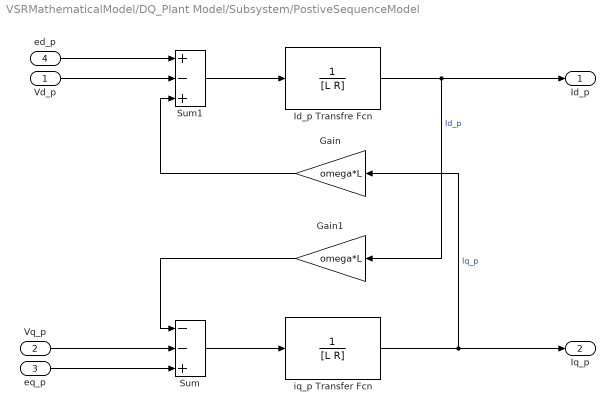
== system VSRMathematicalModel/DQ_Plant Model/Subsystem/PostiveSequenceModel ==
  Vd_p : Inport
  Vq_p : Inport  Port=2
  eq_p : Inport  Port=3
  ed_p : Inport  Port=4
  Gain : Gain  Gain=omega*L
  Gain1 : Gain  Gain=omega*L
  Id_p Transfre Fcn : TransferFcn  Denominator=[L R]
  Sum : Sum  Inputs=--+
  Sum1 : Sum  Inputs=+-+
  iq_p Transfer Fcn : TransferFcn  Denominator=[L R]
  Id_p : Outport
  Iq_p : Outport  Port=2
  wires:
  Vq_p/1 -> Sum/2
  Id_p Transfre Fcn/1 -> Id_p/1, Gain1/1  "Id_p"
  Sum/1 -> iq_p Transfer Fcn/1
  Sum1/1 -> Id_p Transfre Fcn/1
  Gain1/1 -> Sum/1
  Vd_p/1 -> Sum1/2
  eq_p/1 -> Sum/3
  iq_p Transfer Fcn/1 -> Iq_p/1, Gain/1  "Iq_p"
  Gain/1 -> Sum1/3
  ed_p/1 -> Sum1/1

== matlab function VSRMathematicalModel/Subsystem/Vabc//Vdq1 ==
  data: va input; vd output; vb input; vc input; theta input; vq output
function [vd,vq]= fcn(va,vb,vc,theta)

vd = 2/3*(va*cos(theta)+vb*cos(theta-2*pi/3)+vc*cos(theta+2*pi/3));
vq = -2/3*(va*sin(theta)+vb*sin(theta-2*pi/3)+vc*sin(theta+2*pi/3));

== matlab function VSRMathematicalModel/Subsystem/Vabc//Vdq ==
  data: va input; vd output; vb input; vc input; theta input; vq output
function [vd,vq]= fcn(va,vb,vc,theta)

vd = 2/3*(va*cos(theta)+vb*cos(theta-2*pi/3)+vc*cos(theta+2*pi/3));
vq = -2/3*(va*sin(theta)+vb*sin(theta-2*pi/3)+vc*sin(theta+2*pi/3));

== matlab function VSRMathematicalModel/DQ_Plant Model/MATLAB Function ==
  data: Grid_Voltages input; P output; DQ_Current input; theta input; Q output; S output
function [P,Q,S] = fcn(Grid_Voltages,DQ_Current,theta)

% Extract Grid Components
edp = Grid_Voltages(1); eqp = Grid_Voltages(2);
edn = Grid_Voltages(3); eqn = Grid_Voltages(4);

idp = DQ_Current(1); iqp = DQ_Current(2);
idn = DQ_Current(3); iqn = DQ_Current(4);


P0 = 1.5*(edp*idp + eqp*iqp + edn*idn + eqn*iqn);
Pc2 = 1.5*(edp*idn + eqp*iqn + edn*idp + eqn*iqp);
Ps2 = 1.5*(eqn*idp - edn*iqp - eqp*idn + edp*iqn);

Q0 = 1.5*(eqp*idp - edp*iqp + eqn*idn - edn*iqn);
Qc2 = 1.5*(eqp*idn - edp*iqn + eqn*idp - edn*iqp);
Qs2 = 1.5*(edp*idn + eqp*iqn - edn*idp - eqn*iqp);

P = P0 + Pc2*cos(2*theta) + Ps2*sin(2*theta);
Q = Q0 + Qc2*cos(2*theta) + Qs2*sin(2*theta);
S = [P0, Q0, Pc2, Ps2];

== matlab function VSRMathematicalModel/MPC_Controller_V1 ==
  data: Vdc_ref input; i_ref output; Vdc_meas input; Grid_Voltages input; P_load_est input; I_max input
function i_ref  = fcn(Vdc_ref, Vdc_meas, Grid_Voltages, P_load_est, I_max)
% MPC Controller for Active Rectifier (Unbalanced Grid)
% Inputs:
%   Vdc_ref:       Target DC Voltage (V)
%   Vdc_meas:      Measured DC Voltage (V)
%   Grid_Voltages: Vector [Ed_p, Eq_p, Ed_n, Eq_n] from PLL/Seq Separator
%   P_load_est:    Estimated Load Power (W)
%   I_max:         Current Limit (A)
% Output:
%   i_ref:         Vector [id_p; iq_p; id_n; iq_n]

    % --- 1. Setup for Simulink -------------------------------------------
    % Declare 'quadprog' as extrinsic (Simulink will run it in MATLAB engine)
    coder.extrinsic('quad_wright');
    %coder.extrinsic('optimizationset');
    %coder.extrinsic('kron'); % Useful for matrix expansion
    
    % --- 2. System Parameters ---
    % UPDATE: Run MPC 10x slower than Switching Freq (10 kHz)
    Ts    = 5e-04;        % Sampling Time = 1 ms (1 kHz)
    C_dc  = 1500e-6;     % DC Capacitor (F)
    Np    = 30;           % Prediction Horizon (Keep low for speed: 3 to 5)
    u_dim = 4;           % Number of inputs [id_p, iq_p, id_n, iq_n]
    
    % --- 3. Tuning Weights -----------------------------------------------
    lambda_W   = 250;    % Weight on DC Voltage/Energy Tracking
    lambda_Q   = 500;     % Weight on Reactive Power (keep near 0)
    lambda_Rip = 20000;     % Weight on Ripple Suppression (Pc2, Ps2)
    lambda_R   = 2000000;    % Control Effort Penalty (Smoothing)
    
    % --- 4. Matrices Construction ----------------------------------------
    % Extract Grid Components
    Ed_p = Grid_Voltages(1); Eq_p = Grid_Voltages(2);
    Ed_n = Grid_Voltages(3); Eq_n = Grid_Voltages(4);
    
    % G Matrix (Power Coefficients)
    % Rows: [P0; Q0; Pc2; Ps2]
    G = 1.5 * [ Ed_p,  Eq_p,  Ed_n,  Eq_n; ...   
                Eq_p, -Ed_p,  Eq_n, -Ed_n; ...   
                Ed_n,  Eq_n,  Ed_p,  Eq_p; ...   
                Eq_n, -Ed_n, -Eq_p,  Ed_p ];     
            
    % Split dynamics
    G_P = G(1,:);       % Real Power (Affects Energy W)
    G_Aux = G(2:4,:);   % Q and Ripples (To be minimized)
    
    % Discrete State Space for Energy: W(k+1) = W(k) + B*u(k) + D
    B_sys = (2 * Ts / C_dc) * G_P; 
    D_dist = -(2 * Ts / C_dc) * P_load_est;
    
    % --- 5. Prediction Matrices (Lifted System) --------------------------
    % Initialize Su (Input to State) matrix
    % Since A=1, Su is a lower triangular matrix of B_sys blocks
    % Note: Pre-allocating for code generation compatibility
    Su = zeros(Np, Np*u_dim);
    
    % Construct Su manually (simpler than loops for Simulink Coder sometimes)
    % But extrinsic 'kron' or loops are fine for simulation.
    for i = 1:Np
        for j = 1:i
            % Fill blocks: column index for u(k+j-1)
            col_idx = (j-1)*u_dim + 1 : j*u_dim;
            Su(i, col_idx) = B_sys; 
        end
    end
    
    % Sx (Initial State) and Sd (Disturbance)
    Sx = ones(Np, 1);
    Sd = (1:Np)' * D_dist;
    
    % --- 6. QP Problem Formulation ---------------------------------------
    % Current Energy State
    W_k = Vdc_meas^2;
    W_target = Vdc_ref^2;
    W_ref_vec = W_target * ones(Np, 1);
    
    % Constant part of error: (Ref - Sx*W0 - Sd)
    const_part = W_ref_vec - Sx*W_k - Sd;
    
    % Weight Matrices (Expanded for Horizon)
    % We use loops/diag to avoid extrinsic kron issues if possible, 
    % but extrinsic call is safer for rapid prototyping.
    I_np = eye(Np);
    Q_W_big = lambda_W * I_np;
    
    % Aux Weights (Q, Ripple)
    Q_aux_base = diag([lambda_Q, lambda_Rip, lambda_Rip]);
    % Expansion: kron(eye(Np), Q_aux_base)
    % We calculate the G_big term directly: G_big' * Q_big * G_big
    % Since Ripples are instantaneous, this is block diagonal.
    % Term = Sum (G_Aux' * Q_aux_base * G_Aux) for each step
    H_aux_block = G_Aux' * Q_aux_base * G_Aux;
    
    % R Matrix (Regularization)
    R_base = lambda_R * eye(u_dim);
    
    % Construct H (Hessian)
    % H = 2 * (Su' * Q_W * Su + blkdiag(H_aux) + R)
    H_tracking = Su' * Q_W_big * Su;
    
    % Add Aux and R terms to diagonal blocks of H
    H_qp = 2 * H_tracking;
    for k = 1:Np
       idx = (k-1)*u_dim + 1 : k*u_dim;
       H_qp(idx, idx) = H_qp(idx, idx) + 2*(H_aux_block + R_base);
    end

    % Construct f (Linear term)
    % f = -2 * const_part' * Q_W * Su
    f_qp = -2 * const_part' * Q_W_big * Su;
    f_qp = f_qp'; % Transpose to column vector
    
    % Constraints (LB / UB)
    n_vars = Np * u_dim;
    I_all = eye(n_vars);
    A_ineq = [ I_all; -I_all ]; 
    limit_vec = I_max * ones(n_vars, 1);
    b_ineq = [ limit_vec; limit_vec ]; 
    
    % --- 7. Solve Optimization -------------------------------------------
    % Set options for interior-point-convex
    %opts = optimset('Display','off', 'Algorithm','interior-point-convex');
    
    % Call Solver
    % Initialize U_opt to zero in case solver fails
    x0 = zeros(n_vars, 1);
    U_opt = zeros(n_vars, 1);
    U_sol = zeros(n_vars, 1);
    
    [U_sol, ~] = quad_wright(H_qp, f_qp, A_ineq, b_ineq, [], [], x0, []);
    %[U_sol, ~] = quadprog(H_qp, f_qp, [], [], [], [], LB, UB, [], opts);
    
    if ~isempty(U_sol)
        U_opt = U_sol;
    end
    
    % Extract first control step
    i_ref = U_opt(1:u_dim);

end

== matlab function VSRMathematicalModel/PLL1/V_AlphaBeta//Vdq ==
  data: valpha input; vd output; vbeta input; theta input; vq output
function [vd,vq]= fcn(valpha,vbeta,theta)

vd = (valpha*cos(theta)+vbeta*sin(theta));
vq = (-valpha*sin(theta)+vbeta*cos(theta));

== matlab function VSRMathematicalModel/PLL1/Vabc//V_AlphaBeta ==
  data: va input; valpha output; vb input; vc input; vbeta output
function [valpha,vbeta]= fcn(va,vb,vc)

valpha = 2/3*(va - 0.5*vb - 0.5*vc);
vbeta =  2/3*(sqrt(3)/2*vb - sqrt(3)/2*vc);

== matlab function VSRMathematicalModel/PLL1/ctrlGain ==
  data: ed input; gamma1 output; eq input; gamma2 output
function [gamma1,gamma2] = fcn(ed,eq)

phi = 2*pi*100;

eg = sqrt(ed^2+eq^2);

gamma1 = (phi^2)/eg;
gamma2 = (2*phi)/eg;
